simulink model "ACC"  (R2017b)
settings: Solver=ode3  StartTime=0.0  StopTime=inf  FixedStep=0.02  RelTol=1e-3  EnableMultiTasking=on
undefined symbols (not defined in the file or in its folder): control, data
libraries: simulink x11
settings Model: SimulationMode=accelerator  Creator=Owen  LastModifiedBy=alessiotumminello
settings DataIOCC: LimitDataPoints=on  SaveFormat=Array
settings OptimizationCC: LifeSpan=inf  AccelVerboseBuild=on
settings DebuggingCC: SolverPrmCheckMsg=warning  SFUnexpectedBacktrackingDiag=warning  SFNoUnconditionalDefaultTransitionDiag=warning  SFExecutionAtInitializationDiag=none
settings HardwareCC: ProdBitPerPointer=32  ProdBitPerSizeT=32  ProdBitPerPtrDiffT=32  ProdLargestAtomicFloat=None  ProdIntDivRoundTo=Undefined  ProdEndianess=Unspecified  ProdWordSize=32  ProdHWDeviceType=32-bit Generic
settings ModelReferenceCC: PropagateSignalLabelsOutOfModel=off
settings SFSimCC: SimCustomInitializer=initTORCSLink();  SimCustomTerminator=terminateTORCSLink();  SimUserSources=TORCSLink.c  SimBuildMode=sf_nonincremental_build  SimGenImportedTypeDefs=on
settings CodeAppCC: StateflowObjectComments=on
settings GRTTargetCC: TargetLangStandard=C89/C90 (ANSI)  GeneratePreprocessorConditionals=Disable all
settings ConfigComp: CovMetricSettings=dw  CovHtmlReporting=on  CovSaveCumulativeToWorkspaceVar=on  CovSaveSingleToWorkspaceVar=on  CovExternalEMLEnable=off  CovSFcnEnable=off

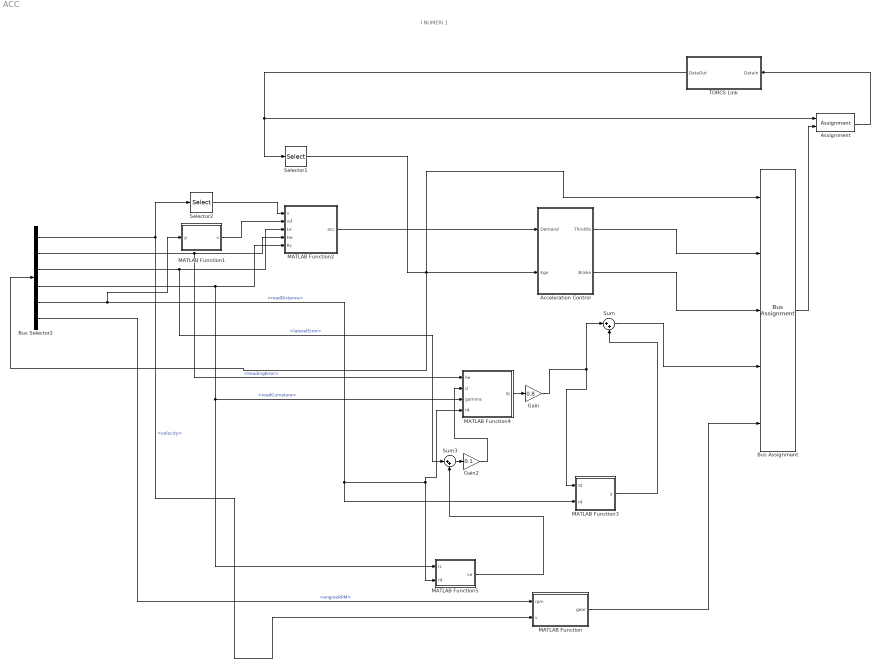
== system ACC ==
  note: I NUMERI 1
  Acceleration Control : Subsystem
  Assignment : Assignment  DiagnosticForDimensions=Warning  IndexOptions=Index vector (dialog)  Indices=1  OutputSizes=1
  Bus Assignment : BusAssignment  AssignedSignals=control.throttle,control.brake,control.steering,control.gear
  Bus Selector2 : BusSelector  OutputSignals=data.velocity,data.headingError,data.lateralError,data.roadCurvature,data.roadDistance,data.engineRPM
  Gain : Gain  Gain=0.8
  Gain2 : Gain  Gain=0.1
  MATLAB Function : MATLAB Function  TreatAsAtomicUnit=on
  MATLAB Function1 : MATLAB Function  TreatAsAtomicUnit=on
  MATLAB Function2 : MATLAB Function  TreatAsAtomicUnit=on
  MATLAB Function3 : MATLAB Function  TreatAsAtomicUnit=on
  MATLAB Function4 : MATLAB Function  TreatAsAtomicUnit=on
  MATLAB Function5 : MATLAB Function  TreatAsAtomicUnit=on
  Selector1 : Selector  InputPortWidth=10  IndexOptions=Index vector (dialog)  Indices=1  OutputSizes=1
  Selector2 : Selector  InputPortWidth=3  IndexOptions=Index vector (dialog)  Indices=1  OutputSizes=1
  Sum : Sum  Inputs=|++
  Sum3 : Sum  Inputs=|++
  TORCS Link : Subsystem  LoadFcn=|  InitFcn=|
      LoadFcn=|
      | load VehicleBusses.mat;
      | src = 'TORCSLink.c';
      | init = 'initTORCSLink();';
      | term = 'terminateTORCSLink();';
      | simSrc = get_param(gcs,'SimUserSources');
      | simInit = get_param(gcs,'SimCustomInitializer');
      | simTerm = get_param(gcs,'SimCustomTerminator');
      | 
      | if isempty(strfind(simSrc,src))
      |   fprintf('Adding %s to Custom Sources\n', src);
      |   set_param(gcs,'SimUserSources', [simSrc 10 src]);
      | end
      | 
      | if isempty(strfind(simInit,init))
      |   fprintf('Adding %s to Custom Initialisation Code\n', init);
      |   set_param(gcs,'SimCustomInitializer', [simInit 10 init]);
      | end
      | 
      | if isempty(strfind(simTerm,term))
      |   fprintf('Adding %s to Custom Termination Code\n', term);
      |   set_param(gcs,'SimCustomTerminator', [simTerm 10 term]);
      | end
      | 
      | if isunix
      |     libs = 'librt.so';
      |     simLibs = get_param(gcs,'SimUserLibraries');
      | 
      |     if isempty(strfind(simLibs,libs))
      |       fprintf('Adding %s to Custom Libraries\n', libs);
      |       set_param(gcs,'SimUserLibraries', [simLibs 10 libs]);
      |     end
      | else
      |    set_param(gcs,'SimUserLibraries', '');
      | end
      | 
      | clear src init term simSrc simInit simTerm libs simLibs;
      InitFcn=|
      | load VehicleBusses.mat;
      | src = 'TORCSLink.c';
      | init = 'initTORCSLink();';
      | term = 'terminateTORCSLink();';
      | simSrc = get_param(gcs,'SimUserSources');
      | simInit = get_param(gcs,'SimCustomInitializer');
      | simTerm = get_param(gcs,'SimCustomTerminator');
      | 
      | if isempty(strfind(simSrc,src))
      |   fprintf('Adding %s to Custom Sources\n', src);
      |   set_param(gcs,'SimUserSources', [simSrc 10 src]);
      | end
      | 
      | if isempty(strfind(simInit,init))
      |   fprintf('Adding %s to Custom Initialisation Code\n', init);
      |   set_param(gcs,'SimCustomInitializer', [simInit 10 init]);
      | end
      | 
      | if isempty(strfind(simTerm,term))
      |   fprintf('Adding %s to Custom Termination Code\n', term);
      |   set_param(gcs,'SimCustomTerminator', [simTerm 10 term]);
      | end
      | 
      | if isunix
      |     libs = 'librt.so';
      |     simLibs = get_param(gcs,'SimUserLibraries');
      | 
      |     if isempty(strfind(simLibs,libs))
      |       fprintf('Adding %s to Custom Libraries\n', libs);
      |       set_param(gcs,'SimUserLibraries', [simLibs 10 libs]);
      |     end
      | else
      |    set_param(gcs,'SimUserLibraries', '');
      | end
      | 
      | clear src init term simSrc simInit simTerm libs simLibs;
  wires:
  Assignment/1 -> TORCS Link/1(DataIn)
  Bus Assignment/1 -> Assignment/2
  TORCS Link/1(DataOut) -> Selector1/1, Assignment/1
  Selector2/1 -> MATLAB Function2/1(v)
  MATLAB Function3/1(y) -> Sum/2
  Sum/1 -> Bus Assignment/4
  Bus Selector2/4 -> MATLAB Function4/3(gamma), MATLAB Function5/1(rc), MATLAB Function2/5(Rc)  "<roadCurvature>"
  Bus Selector2/3 -> Sum3/1, MATLAB Function2/3(Le)  "<lateralError>"
  Gain/1 -> MATLAB Function3/1(St), Sum/1
  Bus Selector2/2 -> MATLAB Function4/1(he), MATLAB Function2/4(He)  "<headingError>"
  Bus Selector2/1 -> Selector2/1, MATLAB Function/2(v)  "<velocity>"
  MATLAB Function/1(gear) -> Bus Assignment/5
  Acceleration Control/1(Throttle) -> Bus Assignment/2
  Acceleration Control/2(Brake) -> Bus Assignment/3
  MATLAB Function2/1(acc) -> Acceleration Control/1(Demand)
  Bus Selector2/6 -> MATLAB Function/1(rpm)  "<engineRPM>"
  Bus Selector2/5 -> MATLAB Function1/1(p), MATLAB Function4/4(rd), MATLAB Function5/2(rd), MATLAB Function3/2(rd)  "<roadDistance>"
  Sum3/1 -> Gain2/1
  Gain2/1 -> MATLAB Function4/2(d)
  MATLAB Function5/1(Le) -> Sum3/2
  MATLAB Function4/1(St) -> Gain/1
  Selector1/1 -> Bus Selector2/1, Bus Assignment/1, Acceleration Control/2(Ego)
  MATLAB Function1/1(v) -> MATLAB Function2/2(vd)

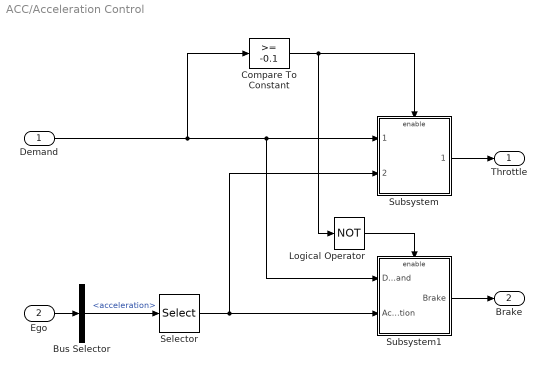
== system ACC/Acceleration Control ==
  Demand : Inport
  Ego : Inport  Port=2
  Bus Selector : BusSelector  OutputSignals=data.acceleration
  Compare To Constant : simulink/Logic and Bit Operations/Compare To Constant  relop=>=  const=-0.1  OutDataTypeStr=boolean
  Logical Operator : Logic  Operator=NOT  AllPortsSameDT=off  OutDataTypeStr=boolean
  Selector : Selector  InputPortWidth=3  IndexOptions=Index vector (dialog)  Indices=1  OutputSizes=1
  Subsystem : Subsystem
  Subsystem1 : Subsystem
  Throttle : Outport
  Brake : Outport  Port=2
  wires:
  Selector/1 -> Subsystem/2(Acceleration), Subsystem1/2(Acceleration)
  Demand/1 -> Compare To Constant/1, Subsystem1/1(Demand), Subsystem/1(Demand)
  Subsystem1/1(Brake) -> Brake/1
  Subsystem/1(Throttle) -> Throttle/1
  Compare To Constant/1 -> Subsystem/Enable, Logical Operator/1
  Logical Operator/1 -> Subsystem1/Enable
  Ego/1 -> Bus Selector/1
  Bus Selector/1 -> Selector/1  "<acceleration>"

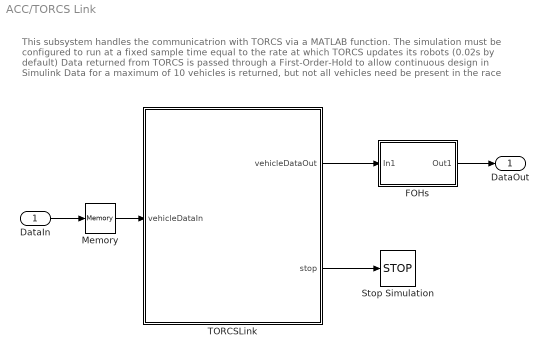
== system ACC/TORCS Link ==
  note: This subsystem handles the communicatrion with TORCS via a MATLAB function.
      | The simulation must be configured to run at a fixed sample time equal to the rate at which TORCS updates its robots (0.02s by default)
      | Data returned from TORCS is passed through a First-Order-Hold to allow continuous design in Simulink
      | Data for a maximum of 10 vehicles is returned, but not all vehicles need be present in the race
  DataIn : Inport
  FOHs : Subsystem  TreatAsAtomicUnit=on
  Memory : Memory
  Stop Simulation : Stop
  TORCSLink : MATLAB Function  TreatAsAtomicUnit=on
  DataOut : Outport
  wires:
  Memory/1 -> TORCSLink/1(vehicleDataIn)
  TORCSLink/1(vehicleDataOut) -> FOHs/1(In1)
  FOHs/1(Out1) -> DataOut/1
  DataIn/1 -> Memory/1
  TORCSLink/2(stop) -> Stop Simulation/1

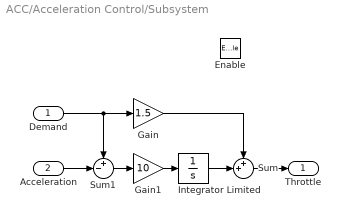
== system ACC/Acceleration Control/Subsystem ==
  Demand : Inport
  Acceleration : Inport  Port=2
  Enable : EnablePort  StatesWhenEnabling=reset
  Gain : Gain  Gain=1.5
  Gain1 : Gain  Gain=10
  Integrator Limited : Integrator  LimitOutput=on  UpperSaturationLimit=1  LowerSaturationLimit=-1
  Sum : Sum  Inputs=++|
  Sum1 : Sum  Inputs=+-|
  Throttle : Outport  OutputWhenDisabled=reset  InitialOutput=0
  wires:
  Gain/1 -> Sum/1
  Integrator Limited/1 -> Sum/2
  Gain1/1 -> Integrator Limited/1
  Sum/1 -> Throttle/1
  Demand/1 -> Sum1/1, Gain/1
  Acceleration/1 -> Sum1/2
  Sum1/1 -> Gain1/1

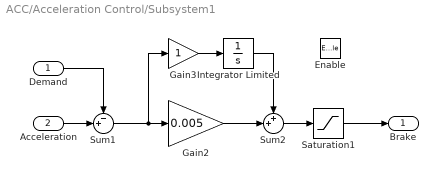
== system ACC/Acceleration Control/Subsystem1 ==
  Demand : Inport
  Acceleration : Inport  Port=2
  Enable : EnablePort  StatesWhenEnabling=reset
  Gain2 : Gain  Gain=0.005
  Gain3 : Gain
  Integrator Limited : Integrator  LimitOutput=on  UpperSaturationLimit=1  LowerSaturationLimit=-1
  Saturation1 : Saturate  UpperLimit=1  LowerLimit=0
  Sum1 : Sum  Inputs=-+|
  Sum2 : Sum  Inputs=++|
  Brake : Outport  OutputWhenDisabled=reset  InitialOutput=0
  wires:
  Sum2/1 -> Saturation1/1
  Gain2/1 -> Sum2/2
  Integrator Limited/1 -> Sum2/1
  Gain3/1 -> Integrator Limited/1
  Sum1/1 -> Gain2/1, Gain3/1
  Demand/1 -> Sum1/1
  Acceleration/1 -> Sum1/2
  Saturation1/1 -> Brake/1

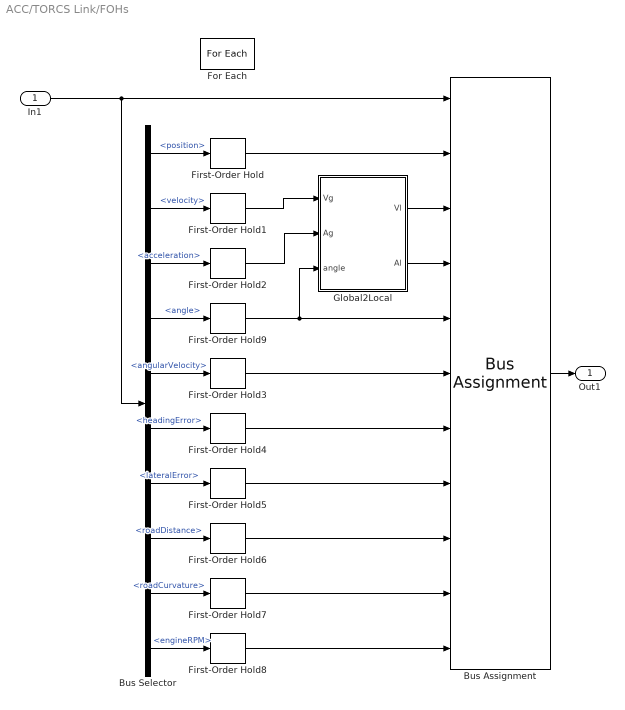
== system ACC/TORCS Link/FOHs ==
  In1 : Inport  Partition=on  PartitionDimension=1  PartitionWidth=1  PartitionOffset=0
  Bus Assignment : BusAssignment  AssignedSignals=data.position,data.velocity,data.acceleration,data.angle,data.angularVelocity,data.headingError,data.lateralError,data.roadDistance,data.roadCurvature,data.engineRPM
  Bus Selector : BusSelector  OutputSignals=data.position,data.velocity,data.acceleration,data.angle,data.angularVelocity,data.headingError,data.lateralError,data.roadDistance,data.roadCurvature,data.engineRPM
  First-Order Hold{,1..9} (10 alike) : simulink/Discrete/First-Order Hold  DisableCoverage=on  Ts=0.02
      settings: SourceProductName=Simulink  SourceProductBaseCode=SL
  For Each : ForEach  DisableCoverage=on  IndexMode=One-based
  Global2Local : MATLAB Function  TreatAsAtomicUnit=on
  Out1 : Outport  ConcatenationDimension=1
  wires:
  Bus Assignment/1 -> Out1/1
  Bus Selector/10 -> First-Order Hold8/1  "<engineRPM>"
  Bus Selector/9 -> First-Order Hold7/1  "<roadCurvature>"
  Bus Selector/8 -> First-Order Hold6/1  "<roadDistance>"
  Bus Selector/7 -> First-Order Hold5/1  "<lateralError>"
  Bus Selector/6 -> First-Order Hold4/1  "<headingError>"
  Bus Selector/5 -> First-Order Hold3/1  "<angularVelocity>"
  Bus Selector/3 -> First-Order Hold2/1  "<acceleration>"
  Bus Selector/2 -> First-Order Hold1/1  "<velocity>"
  Bus Selector/1 -> First-Order Hold/1  "<position>"
  In1/1 -> Bus Assignment/1, Bus Selector/1
  Bus Selector/4 -> First-Order Hold9/1  "<angle>"
  First-Order Hold9/1 -> Global2Local/3(angle), Bus Assignment/5
  First-Order Hold3/1 -> Bus Assignment/6
  First-Order Hold4/1 -> Bus Assignment/7
  First-Order Hold5/1 -> Bus Assignment/8
  First-Order Hold6/1 -> Bus Assignment/9
  First-Order Hold7/1 -> Bus Assignment/10
  First-Order Hold8/1 -> Bus Assignment/11
  First-Order Hold1/1 -> Global2Local/1(Vg)
  First-Order Hold2/1 -> Global2Local/2(Ag)
  First-Order Hold/1 -> Bus Assignment/2
  Global2Local/2(Al) -> Bus Assignment/4
  Global2Local/1(Vl) -> Bus Assignment/3

== matlab function ACC/TORCS Link/TORCSLink ==
  data: vehicleDataIn input Bus: VehicleBus size=10; vehicleDataOut output Bus: VehicleBus size=10; stop output
function [vehicleDataOut, stop] = TORCSLink(vehicleDataIn)
%#codegen
stop = 0;
flag = int32(0);

% Simulink doesn't like passing the array of structures to C function (no
% idea why?!), so we have to seperate out the three stages

% Update vehicle control values in TORCS
for i=1:10
    flag = coder.ceval('setVehicleControl', int32(i-1), vehicleDataIn(i).control);
    if (flag < 0)
        fprintf('No connection to TORCS!\n');
        stop = 1;
    end
end

% Tell TORCS it can update (this function hangs until new data is
% available)
flag = coder.ceval('updateTORCS');
if (flag < 0)
    fprintf('No data from TORCS! (%d) \n', flag);
    stop = 1;
end

% Read in new data from TORCS
for i=1:10
    % Can't pass this directly to coder.ref
    data = vehicleDataIn(i).data;
    flag = coder.ceval('getVehicleData', int32(i-1), coder.ref(data));
    vehicleDataIn(i).data = data;
    if (flag < 0)
        fprintf('No connection to TORCS!\n');
        stop = 1;
    end
end

vehicleDataOut = vehicleDataIn;

== matlab function ACC/TORCS Link/FOHs/Global2Local ==
  data: Vg input; Ag input; angle input; Vl output; Al output
function [Vl,Al] = fcn(Vg,Ag,angle)
%#codegen

phi=angle(3);
R = [cos(phi) sin(phi) 0; -sin(phi) cos(phi) 0; 0 0 1];

Vl = R*Vg;
Al = R*Ag;

== matlab function ACC/MATLAB Function ==
  settings: updateMethod=DISCRETE
  data: rpm input; gear output; v input
function gear  = gear(rpm, v)
%#codegen
statos1=0;
statod1=0;
rpm1=0;
v=v(1);
persistent gear1 statos statod;
if isempty(gear1)
    gear1= int32(1);
    statos = 0;
    statod= 0;
end
if  v<18 && v>0
    gear1=int32(1);
end
if  v>18 && v<27
    gear1=int32(2);
end

if rpm < 16000
    statos =1;
end
if rpm > 9500
    statod =1;
end
    
if  rpm > 16000 && statos == 1 && gear1<7 && gear1>1
    gear1= gear1+1;
    statos=0;
end
if rpm<9500 && statod == 1 && gear1>2
    gear1= gear1-1;
    statod=0;
end

gear = gear1;

== matlab function ACC/MATLAB Function4 ==
  data: he input; St output; d input; gamma input; rd input
function St = sterzo(he, d, gamma,rd)
%#codegen
k=2.8;
he=-he;
St= (-k*he- d*sinc(he) + (cos(he)*gamma/(1-d*gamma)))*0.5;
if St < -0.785398
    St=-0.785398;
elseif St > 0.785398
     St=0.785398;   
end
St=St/0.785398;
if rd>2635 && rd<2820
 if St < -0.9
    St=-0.9;
elseif St > 0.9
     St=0.9; 
 end
else  
if St < -0.6
    St=-0.6;
elseif St > 0.6
     St=0.6;   
end
 end

== matlab function ACC/MATLAB Function5 ==
  data: rc input; Le output; rd input
function Le = fcn(rc, rd)
if rd>0 && rd<100
    Le=-4.3;
elseif rd>100 && rd<325
    Le=-4.3;
elseif rd>450 && rd<508
    Le=-1 ;
elseif rd>1907 && rd<2069
    Le=-4.3;
elseif rd>2069 && rd<2140
    Le= 4.3;
elseif rd> 2140 && rd<2220
    Le= -4.3;
elseif rd>2220 && rd<2300
    Le=4.3
elseif rd>2300 && rd<2590
    Le=-4.3
elseif rd>2590 && rd<2720
    Le=3.7
elseif rd>2720 && rd<2825
    Le=-4.3
elseif rd>4985 && rd<5346
    Le=-4.3;
elseif rd>5346 && rd<5420
    Le=4.3;
elseif rd>5420 && rd<5502
    Le=-4.3;
elseif rd>5502 && rd<5606
    Le=4.3;
else
if rc>1.4e-3
    Le=-4.3;
elseif rc<-1.4e-3
    Le=4.3
else Le=0
end
end

%{
if rd>0 && rd<100
    Le=0;
elseif rd>100 && rd<325
    Le=-4.3;
elseif rd>325 && rd<440
    Le=4.3;
elseif rd>440 && rd<520
    Le=0;
elseif rd>520 && rd<630
    Le=4.3
elseif rd>590
    Le=-4.3;
    %}
end

== matlab function ACC/MATLAB Function1 ==
  settings: updateMethod=DISCRETE
  data: p input; v output
function v = speedemand(p)
%#codegen

persistent v1 ;
if isempty(v1)
    v1=7;
end
if p>40 && p<80
    v1=45;
end
if p>80 && p<150
    v1=85;
end

if p>318 && p<330
    v1=53;
end

if p>475 && p<515
    v1=33;
end

if p>580 && p<910
    v1=60;
end

if p>910 && p<1080
    v1=37;
end

if p>1080 && p<1223
    v1=64;
end

if p>1223 && p<1470
    v1=46;
end

if p>1430 && p<1950
    v1=80;
end

if p>1950 && p<2070
    v1=45;
end

if p>2190 && p<2290
    v1=25;
end
if p>2320 && p<2320
    v1=30;
end

if p>2320 && p<2635
    v1=63;
end

if p>2635 && p<2700
    v1=19;
end

if p>2830 && p<2835
    v1=25;
end

if p>2835 && p<3500
    v1=90;
end

if p>3580 && p<3690
    v1=45;
end

if p>4000 && p<5150
    v1=100;
end

if p>5200 && p<5250
    v1=48;
end

if p>5470 
    v1=100;
end

v = v1;

== matlab function ACC/MATLAB Function2 ==
  data: v input; acc output; vd input; Le input; He input; Rc input
function acc = fcn(v, vd, Le, He, Rc)
    Kv=2;
    acc = -Kv*(v-vd)-Le*sin(He)+Rc*He*cos(He)/(1-Le*Rc);
    if acc > 8
        acc=8;
    elseif acc <-14
        acc=-14;
    end
end

== matlab function ACC/MATLAB Function3 ==
  data: St input; y output; rd input
function y = fcn(St, rd)
if rd>2670 && rd<2680
    St=-1;
end

y = St;
